simulink model "model2_panelMotor"  (R2019b)
settings: Solver=VariableStepAuto  StartTime=0.0  StopTime=10.0  RelTol=1e-3
PreLoadFcn:
  | % Set physical parameters
  | panelMotorParams;
values from neighbouring files (symbols this model uses):
  J = m/12*(l^2*cos(beta)^2+d^2*sin(beta)^2+w^2)    [panelMotorParams.m]
  Kd = 5    [panelMotorParams.m]
  Kf = 0.07    [panelMotorParams.m]
  Kg = 2000    [panelMotorParams.m]
  Kt = 0.07    [panelMotorParams.m]
  L = 1e-5    (= 1e-05)    [panelMotorParams.m]
  R = 10    [panelMotorParams.m]
settings Model: Creator=bneiswan  LastModifiedBy=bneiswan

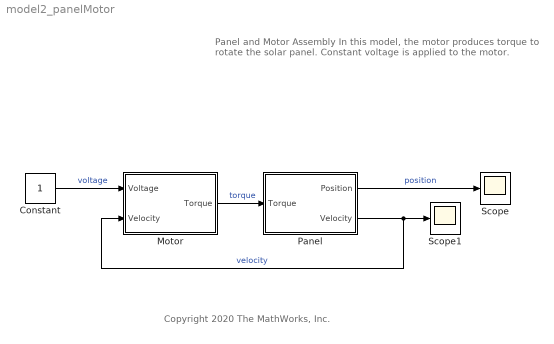
== system model2_panelMotor ==
  note: Copyright 2020 The MathWorks, Inc.
  note: Panel and Motor Assembly
      |
      | In this model, the motor produces torque to rotate the solar panel. Constant voltage is applied to the motor.
  Constant : Constant
  Motor : Subsystem
  Panel : Subsystem
  Scope : Scope
  Scope1 : Scope
  wires:
  Constant/1 -> Motor/1(Voltage)  "voltage"
  Panel/2(Velocity) -> Motor/2(Velocity), Scope1/1  "velocity"
  Motor/1(Torque) -> Panel/1(Torque)  "torque"
  Panel/1(Position) -> Scope/1  "position"

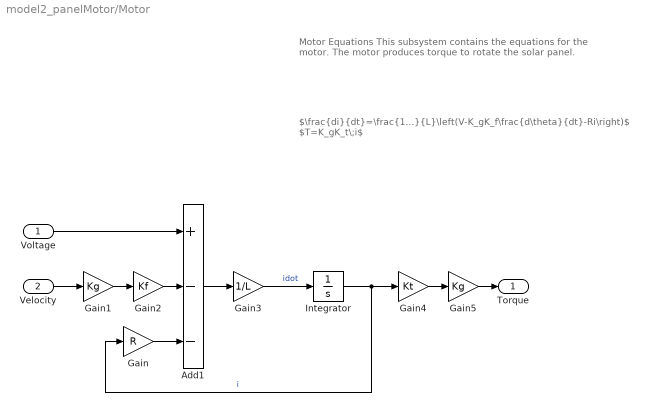
== system model2_panelMotor/Motor ==
  note: $\frac{di}{dt}=\frac{1}{L}\left(V-K_gK_f\frac{d\theta}{dt}-Ri\right)$
      | $T=K_gK_t\;i$
  note: Motor Equations
      |
      | This subsystem contains the equations for the motor. The motor produces torque to rotate the solar panel.
  Voltage : Inport
  Velocity : Inport  Port=2
  Add1 : Sum  Inputs=+--
  Gain : Gain  Gain=R
  Gain1 : Gain  Gain=Kg
  Gain2 : Gain  Gain=Kf
  Gain3 : Gain  Gain=1/L
  Gain4 : Gain  Gain=Kt
  Gain5 : Gain  Gain=Kg
  Integrator : Integrator
  Torque : Outport
  wires:
  Voltage/1 -> Add1/1
  Gain2/1 -> Add1/2
  Gain3/1 -> Integrator/1  "idot"
  Gain/1 -> Add1/3
  Integrator/1 -> Gain4/1, Gain/1  "i"
  Add1/1 -> Gain3/1
  Velocity/1 -> Gain1/1
  Gain4/1 -> Gain5/1
  Gain1/1 -> Gain2/1
  Gain5/1 -> Torque/1

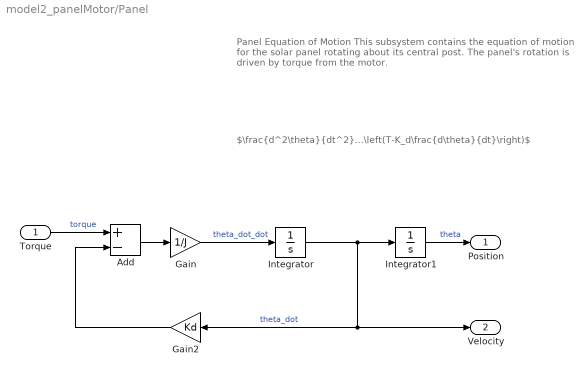
== system model2_panelMotor/Panel ==
  note: $\frac{d^2\theta}{dt^2}=\frac{1}{J}\left(T-K_d\frac{d\theta}{dt}\right)$
  note: Panel Equation of Motion
      |
      | This subsystem contains the equation of motion for the solar panel rotating about its central post. The panel's rotation is driven by torque from the motor.
  Torque : Inport
  Add : Sum  Inputs=+-
  Gain : Gain  Gain=1/J
  Gain2 : Gain  Gain=Kd
  Integrator : Integrator
  Integrator1 : Integrator
  Position : Outport
  Velocity : Outport  Port=2
  wires:
  Torque/1 -> Add/1  "torque"
  Add/1 -> Gain/1
  Integrator/1 -> Integrator1/1, Velocity/1, Gain2/1  "theta_dot"
  Gain2/1 -> Add/2
  Gain/1 -> Integrator/1  "theta_dot_dot"
  Integrator1/1 -> Position/1  "theta"
